simulink model "compute_average_17a"  (R2017a)
settings: Solver=FixedStepAuto  StartTime=0.0  StopTime=12  FixedStep=1  RelTol=1e-3
undefined symbols (not defined in the file or in its folder): sigbuilder_block
settings Model: Creator=wentaodu  LastModifiedBy=wentaodu

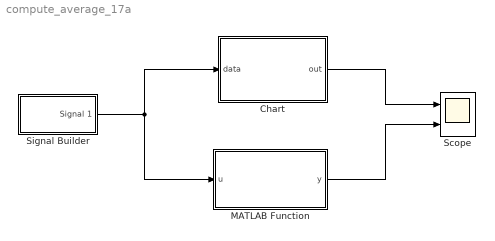
== system compute_average_17a ==
  Chart : Stateflow chart  TreatAsAtomicUnit=on
  MATLAB Function : MATLAB Function  TreatAsAtomicUnit=on
  Scope : Scope  NumInputPorts=2
  Signal Builder : Subsystem  Tag=STV Subsys  LoadFcn=sigbuilder_block('load');  StartFcn=sigbuilder_block('start');  StopFcn=sigbuilder_block('stop');  ClipboardFcn=sigbuilder_block('clipboard');  mask(Sigbuilder block){tuvar=[0:10]}
      mask help: Simulink:masks:SigbuilderBlock_MD
      mask init:
      | if ~strcmp(get_param(bdroot(gcbh),'SimulationStatus'),'stopped') tuvar = sigbuilder_block('maskInit'); end
      settings: CopyFcn=sigbuilder_block('copy');  DeleteFcn=sigbuilder_block('delete');  ModelCloseFcn=sigbuilder_block('modelClose');  PreSaveFcn=sigbuilder_block('preSave');  PauseFcn=sigbuilder_block('pause');  ContinueFcn=sigbuilder_block('continue');  NameChangeFcn=sigbuilder_block('namechange');  OpenFcn=sigbuilder_block('open',[277.5 147.75 550.5 399.75 ]);  CloseFcn=sigbuilder_block('close');
      mask Display: plot(0, 0, 100, 100,[2, 2, 32, 32, 2], [68, 8, 8, 68, 68],[32, 2], [38, 38], [32, 19, 2],[53, 60, 44], [32, 17, 17, 2],[16, 16, 31, 31]);txt = getActiveGroup(gcbh);text(2, 100, txt,'verticalAlignment', 'top');
  wires:
  Signal Builder/1(Signal 1) -> MATLAB Function/1(u), Chart/1(data)
  Chart/1(out) -> Scope/1
  MATLAB Function/1(y) -> Scope/2

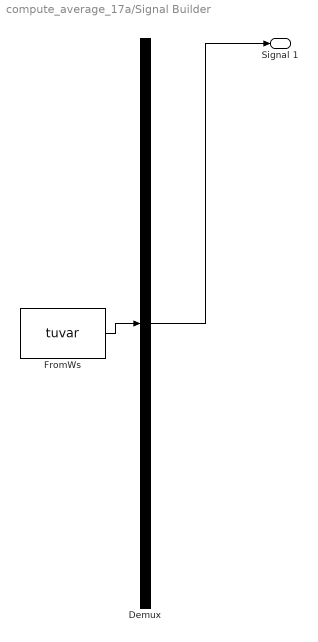
== system compute_average_17a/Signal Builder ==
  Demux : Demux  Tag=STV Demux  Outputs=1
  FromWs : FromWorkspace  Tag=STV FromWs  VariableName=tuvar  SampleTime=0
      SigBuilderData=|
      | common.afterFinalStr = 'Extrapolate'
      | common.sampleTime = 0
      | dataSet.timeRange = [0 10]
      | dataSet.name = 'Group 1'
      | sbobj.Groups.Name = 'Group 1'
      | sbobj.Groups.Signals.Name = 'Signal 1'
      | sbobj.Groups.Signals.XData = [0 3 3 6 6 10]
      | sbobj.Groups.Signals.YData = [0 0 1 1 0 0]
  Signal 1 : Outport  Tag=STV Outport
  wires:
  Demux/1 -> Signal 1/1
  FromWs/1 -> Demux/1

== matlab function compute_average_17a/MATLAB Function ==
  data: u input; y output
function y = compute_average(u)

% Declare two persistent variables
persistent sum cnt

% Initialize the variables
if isempty(sum)
    sum = 0;
    cnt = 0;
end

% Compute the accumulated sum and the number of values so far.
sum = sum + u;
cnt = cnt + 1;

% Return the average for every 4 numbers
if mod(cnt,4)==0
    y = sum/4;
    sum = 0;
else 
    y = 0;
end

== matlab function compute_average_17a/Chart ==
  data: x function_input; y function_output; data input; out output
function y = compute_average(x)

% Declare two persistent variables
persistent sum cnt

% Initialize the variables
if isempty(sum)
    sum = 0;
    cnt = 0;
end

% Compute the accumulated sum and the number of values so far.
sum = sum + x;
cnt = cnt + 1;

% Return the average for every 4 numbers
if mod(cnt,4)==0
    y = sum/4;
    sum = 0;
else
    y = 0;
end
